simulink model "FinalProject"  (R2019a)
settings: Solver=ode3  StartTime=0.0  StopTime=20  RelTol=1e-3  EnableMultiTasking=on
libraries: raspberrypilib x2, embdlinuxlib x1
settings Model: FPTRunName=Active  ExtModeTrigDuration=2  Creator=justindemus  LastModifiedBy=justindemus
settings SolverCC: PositivePriorityOrder=on
settings DataIOCC: LimitDataPoints=on  SaveFormat=Array
settings OptimizationCC: ExpressionDepthLimit=2147483647  LifeSpan=Inf  MaxStackSize=64
settings DebuggingCC: UnderspecifiedInitializationDetection=Classic  MergeDetectMultiDrivingBlocksExec=none  FcnCallInpInsideContextMsg=warning  AllowSymbolicDim=off  StateNameClashWarn=warning  SFUnexpectedBacktrackingDiag=warning  SFNoUnconditionalDefaultTransitionDiag=warning  SFExecutionAtInitializationDiag=none  ArithmeticOperatorsInVariantConditions=warning
settings HardwareCC: ProdBitPerPointer=32  ProdBitPerSizeT=32  ProdBitPerPtrDiffT=32  ProdLargestAtomicInteger=Long  ProdLargestAtomicFloat=Double  ProdWordSize=32  ProdHWDeviceType=ARM Compatible->ARM Cortex  UseEmbeddedCoderFeatures=off
settings ModelReferenceCC: PropagateSignalLabelsOutOfModel=off
settings SFSimCC: SimUseLocalCustomCode=off
settings RTWCC: SystemTargetFile=ert.tlc  HardwareBoard=Raspberry Pi  TemplateMakefile=ert_default_tmf  GenerateReport=on  RTWVerbose=off  RTWUseLocalCustomCode=off  Toolchain=GNU GCC Raspberry Pi  BuildConfiguration=Faster Runs  LaunchReport=on
settings CodeAppCC: ForceParamTrailComments=on  OperatorAnnotations=on  StateflowObjectComments=on  MATLABSourceComments=on
settings ERTTargetCC: MultiwordLength=2048  ERTCustomFileBanners=off  SupportContinuousTime=on  SupportNonInlinedSFcns=on  RemoveResetFunc=off  SupportVariableSizeSignals=on  ModelStepFunctionPrototypeControlCompliant=off
settings ConfigComp: CovMetricSettings=dw  CovHtmlReporting=on  CovSaveCumulativeToWorkspaceVar=on  CovSaveSingleToWorkspaceVar=on  CovExternalEMLEnable=off  CovSFcnEnable=off

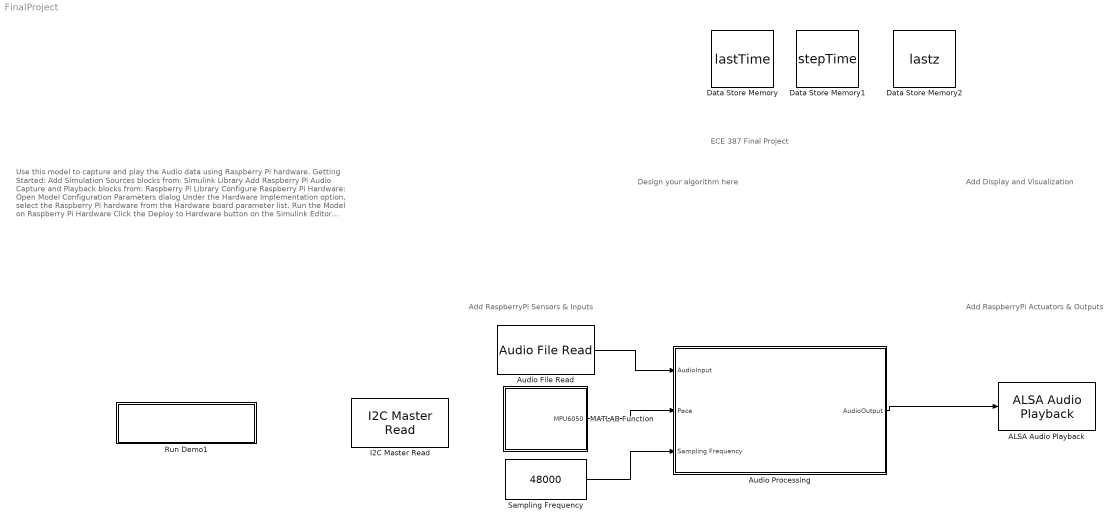
== system FinalProject ==
  note: Use this model to capture and play the Audio data using Raspberry Pi hardware.
      |
      | Getting Started:
      |
      | Add Simulation Sources blocks from:
      | Simulink Library
      | Add Raspberry Pi Audio Capture and Playback blocks from:
      | Raspberry Pi Library
      |
      | Configure Raspberry Pi Hardware:
      |
      | Open Model Configuration Parameters dialog
      | Under the Hardware Implementation option, select the Raspberry Pi hardware from the Hardware board parameter list.
      |
      | Run the Model on Raspberry Pi Hardware
      |
      | Click the Deploy to Hardware button on the Simulink Editor toolbar.
      |
      | Learn More
      | ALSA Audio Capture
      | ALSA Audio Playback
  note: Add Display and Visualization
  note: Design your algorithm here
  note: Add RaspberryPi Actuators & Outputs
  note: ECE 387 Final Project
  note: Add RaspberryPi Sensors & Inputs
  ALSA Audio Playback : embdlinuxlib/ALSA Audio Playback  deviceStr='hw:0,0'  sampleRateEnum=44800  queueDuration=0.5  blockPlatform=Raspberry Pi
      settings: SourceProductName=Simulink Coder Support Package for BeagleBone Blue Hardware  SourceProductBaseCode=SC_BEAGLEBONE_BLUE
  Audio File Read : raspberrypilib/Audio File Read  FileName=guitartune.wav  PlayCount=Inf  OutputEOFIndicator=off  SamplesPerFrame=4410
      settings: SourceProductName=Simulink Support Package for Raspberry Pi Hardware  SourceProductBaseCode=RASPPI
  Audio Processing : Subsystem
  Data Store Memory : DataStoreMemory  DataStoreName=lastTime  ReadBeforeWriteMsg=warning  WriteAfterWriteMsg=warning  WriteAfterReadMsg=warning  ShowAdditionalParam=off  OutDataTypeStr=double
  Data Store Memory1 : DataStoreMemory  DataStoreName=stepTime  ReadBeforeWriteMsg=warning  WriteAfterWriteMsg=warning  WriteAfterReadMsg=warning  ShowAdditionalParam=off  OutDataTypeStr=double
  Data Store Memory2 : DataStoreMemory  DataStoreName=lastz  ReadBeforeWriteMsg=warning  WriteAfterWriteMsg=warning  WriteAfterReadMsg=warning  ShowAdditionalParam=off  OutDataTypeStr=double
  I2C Master Read : raspberrypilib/I2C Master Read  BoardProperty=Pi 3 Model B  Mode=Master  SlaveAddress=10  SlaveByteOrder=BigEndian  Direction=Receiver  RegisterAddressMode=on  RegisterAddress=0  SlaveDataType=uint8  DataLength=1  NoAck=off  RepeatedStart=off  OutputStatus=off  SampleTime=0.1
      settings: SourceProductName=Simulink Support Package for Raspberry Pi Hardware  SourceProductBaseCode=RASPPI
  MATLAB Function : MATLAB Function  TreatAsAtomicUnit=on
  Run Demo1 : Subsystem  Description=Controls host-side RTDX processing.
      mask Display: pic=imread('raspberrypiDeploytoHardware.png');image(pic);
  Sampling Frequency : Constant  Value=48000
  wires:
  Audio File Read/1 -> Audio Processing/1(AudioInput)
  Audio Processing/1(AudioOutput) -> ALSA Audio Playback/1
  Sampling Frequency/1 -> Audio Processing/3(Sampling Frequency)
  MATLAB Function/1(MPU6050) -> Audio Processing/2(Pace)

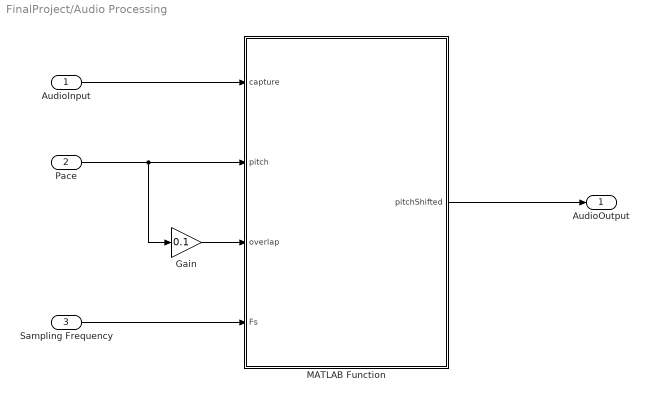
== system FinalProject/Audio Processing ==
  AudioInput : Inport
  Pace : Inport  Port=2
  Sampling Frequency : Inport  Port=3
  "Gain " : Gain  Gain=0.1
  MATLAB Function : MATLAB Function  TreatAsAtomicUnit=on
  AudioOutput : Outport
  wires:
  AudioInput/1 -> MATLAB Function/1(capture)
  MATLAB Function/1(pitchShifted) -> AudioOutput/1
  Pace/1 -> "Gain "/1, MATLAB Function/2(pitch)
  "Gain "/1 -> MATLAB Function/3(overlap)
  Sampling Frequency/1 -> MATLAB Function/4(Fs)

== system FinalProject/Run Demo1 ==

== matlab function FinalProject/MATLAB Function ==
  data lastTime settings: updateMethod=SF_CONTINUOUS_TIME_DATA
  data: MPU6050 output double; lastTime data_store_memory; lastz data_store_memory; stepTime data_store_memory
function MPU6050  = fcn
    rpi = raspi;
    mpu6050 = raspi.internal.mpu6050(rpi, 'i2c-1');
    
    global larErstTime;
    global stepTime;
    global lastz;
    [~,~,z] = readAcceleration(mpu6050);
    if z<0 && lastz==1
        lastz = 0;
        lastTime = tic;
    elseif z>0 && lastz==0
        lastz = 1;
        elapsedTime = toc(lastTime);
        if(elapsedTime/0.6 - 1 <= 0)
            stepTime = 0;
        else
            stepTime = elapsedTime/0.6 - 1;
        end
    end
    MPU6050 = stepTime;
end

== matlab function FinalProject/Audio Processing/MATLAB Function ==
  data: capture input; pitchShifted output; pitch input; overlap input; Fs input
function pitchShifted = pitchShift(capture, pitch, overlap, Fs)

resetFlag = 0;

persistent pitchShifter
if isempty(pitchShifter)
    pitchShifter = audiopluginexample.PitchShifter( ...
        'PitchShift',8,'Overlap',0.3);
    setSampleRate(pitchShifter,Fs);
end

pitchShifted = zeros(size(double(capture)),'like',double(capture));

if nargin > 4 && resetFlag
    reset(pitchShifter);
    return;
end

pitchShifter.PitchShift = pitch;
pitchShifter.Overlap = overlap;

[pitchShifted] = pitchShifter(double(capture));

end
